simulink model "gyroDigControlDemod"  (R2021b)
settings: Solver=FixedStepAuto  StartTime=0.0  StopTime=final_time  FixedStep=step_time  RelTol=1e-3
values from neighbouring files (symbols this model uses):
  ang_vel = ang_vel*pi/180    (= 0.174532925199)    [gyroControlDemod.m]    (also in gyroControlPhaseUnmod.m; gyroDigControlDemod.m; gyroModulationsExample.m = 0.314159265359; gyroSakajiri2008.m)
  I0 = 1    [gyroControlDemod.m]    (also in gyroControlPhaseUnmod.m; gyroDigControlDemod.m; gyroModulationsExample.m; gyroSakajiri2008.m)
  mod_sf = pi/mod_vpi    (= 0.897597901026)    [gyroControlDemod.m]    (also in gyroControlPhaseUnmod.m; gyroDigControlDemod.m; gyroModulationsExample.m; gyroSakajiri2008.m)
  pd_resp = 1    [gyroControlDemod.m]    (also in gyroControlPhaseUnmod.m; gyroDigControlDemod.m; gyroModulationsExample.m; gyroSakajiri2008.m)
  sf = 2*pi*L*D/(lambda*c)    [gyroControlDemod.m]    (also in gyroControlPhaseUnmod.m; gyroDigControlDemod.m; gyroModulationsExample.m; gyroSakajiri2008.m)
  step_time = tau/10    (= 4.58549932353e-07)    [gyroControlDemod.m]    (also in gyroControlPhaseUnmod.m = 2.29274966176e-06; gyroDigControlDemod.m = 2.29274966176e-06; gyroModulationsExample.m = 4.58549932353e-08; gyroSakajiri2008.m = 1.14637483088e-07)
  tau = L/v    (= 4.58549932353e-06)    [gyroControlDemod.m]    (also in gyroControlPhaseUnmod.m; gyroDigControlDemod.m; gyroModulationsExample.m; gyroSakajiri2008.m)
libraries: simulink x1
settings Model: Creator=Stinky  LastModifiedBy=Stinky
settings SolverCC: AlgebraicLoopSolver=TrustRegion
settings DebuggingCC: SFMachineParentedDataDiag=warning

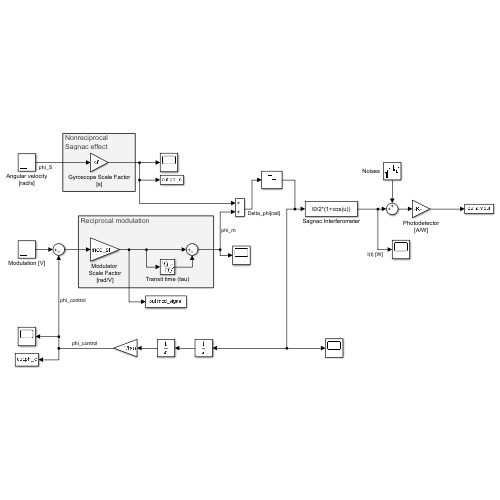
[thumbnail: Simulink's stored preview of the top-level diagram]
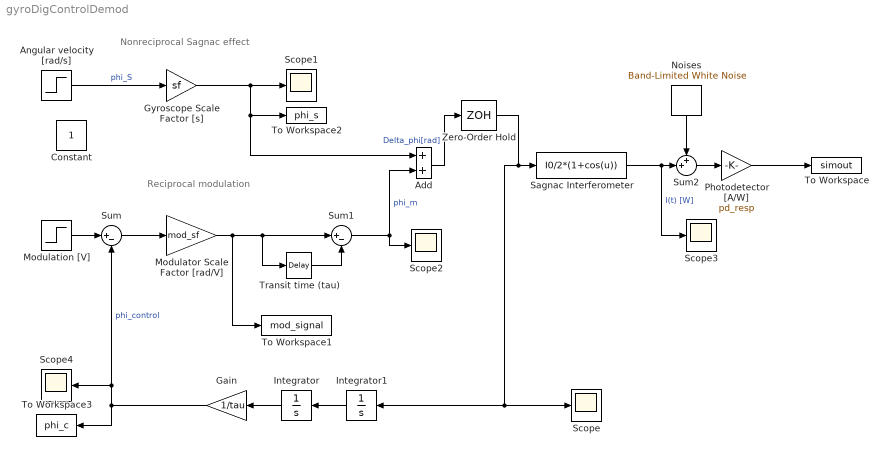
== system gyroDigControlDemod ==
  note: Reciprocal modulation
  note: Nonreciprocal
      | Sagnac effect
  Add : Sum
  Angular velocity [rad/s] : Step  Time=tau  After=ang_vel  SampleTime=0
  Gain : Gain  Gain=1/tau
  Gyroscope Scale Factor [s] : Gain  Gain=sf
  Integrator : Integrator
  Integrator1 : Integrator
  Modulation [V] : Step  Time=0  After=0  SampleTime=0
  Modulator Scale Factor [rad/V] : Gain  Gain=mod_sf
  Noises : simulink/Sources/Band-Limited White Noise  Cov=1e-14  Ts=step_time  seed=[23341]
  Photodetector [A/W] : Gain  Gain=pd_resp
  Sagnac Interferometer : Fcn  Expr=I0/2*(1+cos(u))
  Scope{,1..4} (5 alike) : Scope
  Sum : Sum  Inputs=|+-
  Sum1 : Sum  Inputs=|+-
  Sum2 : Sum  Inputs=++|
  To Workspace : ToWorkspace  VariableName=simout  SaveFormat=Timeseries  SampleTime=-1
  To Workspace1 : ToWorkspace  VariableName=mod_signal  SaveFormat=Timeseries  SampleTime=-1
  To Workspace2 : ToWorkspace  VariableName=phi_s  SaveFormat=Timeseries  SampleTime=-1
  To Workspace3 : ToWorkspace  VariableName=phi_c  SaveFormat=Timeseries  SampleTime=-1
  Transit time (tau) : TransportDelay  DelayTime=tau
  Zero-Order Hold : ZeroOrderHold  SampleTime=-1
  Constant : Constant  IOType=siggen
  wires:
  Transit time (tau)/1 -> Sum1/2
  Sum1/1 -> Scope2/1, Add/2  "phi_m"
  Sum/1 -> Modulator Scale Factor [rad/V]/1
  Photodetector [A/W]/1 -> To Workspace/1
  Sum2/1 -> Photodetector [A/W]/1
  Sagnac Interferometer/1 -> Scope3/1, Sum2/2  "I(t) [W]"
  Noises/1 -> Sum2/1
  Modulation [V]/1 -> Sum/1
  Angular velocity [rad/s]/1 -> Gyroscope Scale Factor [s]/1  "phi_S"
  Integrator/1 -> Gain/1
  Gain/1 -> Scope4/1, Sum/2, To Workspace3/1  "phi_control"
  Integrator1/1 -> Integrator/1
  Gyroscope Scale Factor [s]/1 -> Scope1/1, To Workspace2/1, Add/1
  Modulator Scale Factor [rad/V]/1 -> Sum1/1, Transit time (tau)/1, To Workspace1/1
  Zero-Order Hold/1 -> Integrator1/1, Scope/1, Sagnac Interferometer/1
  Add/1 -> Zero-Order Hold/1  "Delta_phi[rad]"
